simulink model "UAV_Hover_Sim"  (R2025a)
settings: Solver=VariableStepAuto  StartTime=0.0  StopTime=inf  RelTol=1e-3
undefined symbols (not defined in the file): quad_m, W
libraries: aerolibanimutils x1, uavutilslib x1
settings Model: Creator=Aorus PC  LastModifiedBy=esmithzb
settings OptimizationCC: ReuseModelBlockBuffer=off
settings DebuggingCC: UnderspecifiedInitializationDetection=Classic  MergeDetectMultiDrivingBlocksExec=none
settings ModelReferenceCC: PropagateSignalLabelsOutOfModel=off
settings RTWCC: GPUComputeCapability=3.5

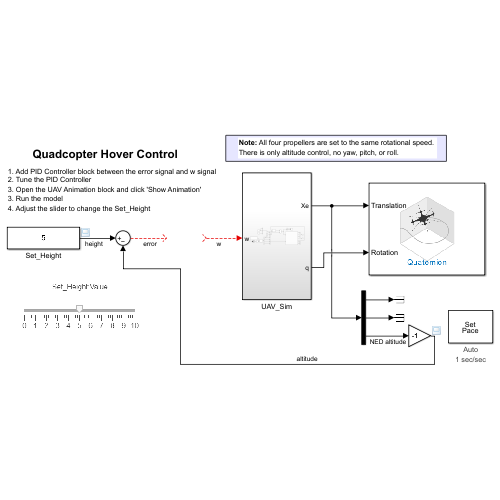
[thumbnail: Simulink's stored preview of the top-level diagram]
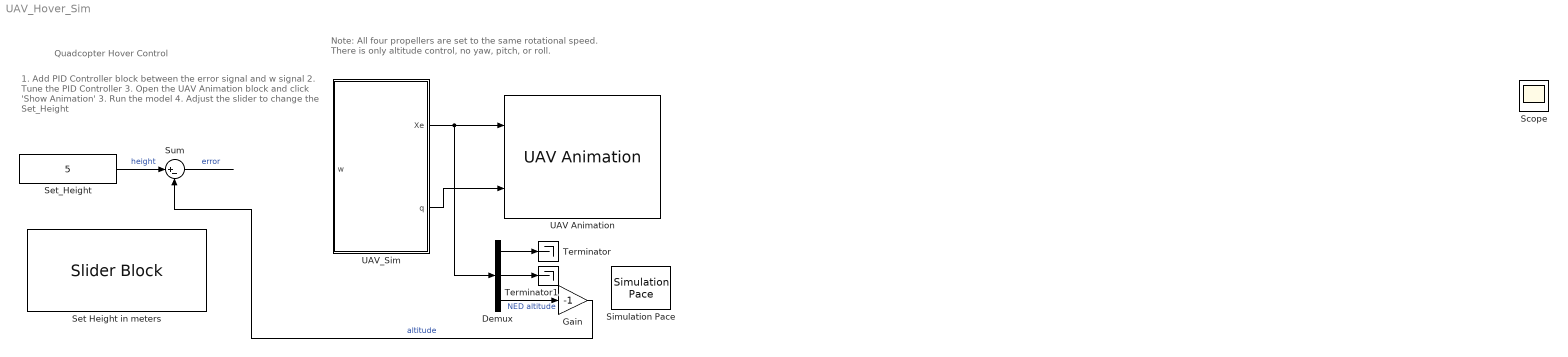
== system UAV_Hover_Sim ==
  note: Note: All four propellers are set to the same rotational speed.
      | There is only altitude control, no yaw, pitch, or roll.
  note: 1. Add PID Controller block between the error signal and w signal 2. Tune the PID Controller
      | 3. Open the UAV Animation block and click 'Show Animation'
      | 3. Run the model
      | 4. Adjust the slider to change the Set_Height
  note: Quadcopter Hover Control
  Demux : Demux  Outputs=3
  Gain : Gain  Gain=-1
  Set Height in meters : SliderBlock  ScaleMax=10  TickInterval=1
  Set_Height : Constant  Value=5
  Simulation Pace : aerolibanimutils/Simulation Pace  SimulationPace=1  SleepMode=Auto  OutputPaceError=off  SampleTime=1/30
  Sum : Sum  Inputs=|+-
  Terminator : Terminator
  Terminator1 : Terminator
  UAV Animation : uavutilslib/UAV Animation  NumUAV=1  DynamicUAVConfig=off  UAVType=Multirotor  UAVSize=4  UAVColor=[1 0 0]  UAVTrajectoryAlpha=1  InertialZDirection=Down  RotationFormat=Quaternion  DrawMarkers=off  SampleTime=-1
  UAV_Sim : Subsystem
  Scope : Scope
      settings: TimeSpan=20  ActiveDisplayYMinimum=0  ActiveDisplayYMaximum=12  YLabel=Altitude (m)
  wires:
  UAV_Sim/1(Xe) -> Demux/1, UAV Animation/1
  UAV_Sim/2(q) -> UAV Animation/2
  Demux/1 -> Terminator/1
  Demux/2 -> Terminator1/1
  Gain/1 -> Sum/2  "altitude"
  Set_Height/1 -> Sum/1  "height"
  Demux/3 -> Gain/1  "NED altitude"
  ? -> UAV_Sim/1(w)  "w"
  Sum/1 -> ?  "error"

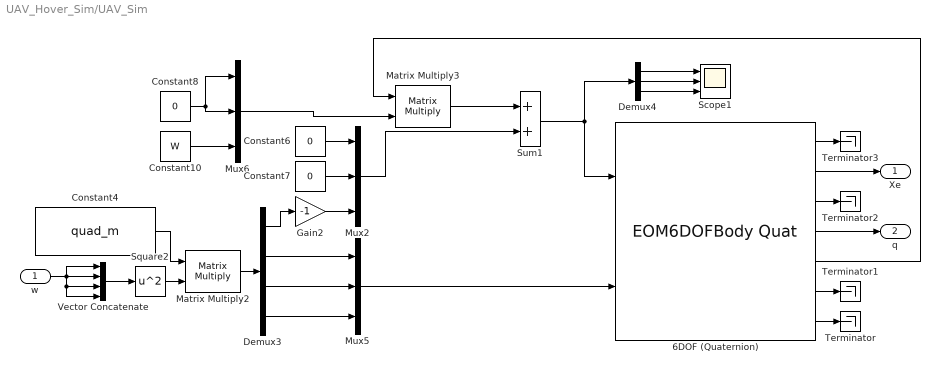
== system UAV_Hover_Sim/UAV_Sim ==
  w : Inport
  6DOF (Quaternion) : EOM6DOFBodyQuat
  Constant10 : Constant  Value=W
  Constant4 : Constant  Value=quad_m
  Constant6 : Constant  Value=0
  Constant7 : Constant  Value=0
  Constant8 : Constant  Value=0
  Demux3 : Demux
  Demux4 : Demux  Outputs=3
  Gain2 : Gain  Gain=-1
  Matrix Multiply2 : Product  Multiplication=Matrix(*)
  Matrix Multiply3 : Product  Multiplication=Matrix(*)
  Mux2 : Mux  Inputs=3
  Mux5 : Mux  Inputs=3
  Mux6 : Mux  Inputs=3
  Scope1 : Scope  NumInputPorts=3
      settings: ActiveDisplayYMinimum=-7E-15  ActiveDisplayYMaximum=8E-16  DataLoggingVariableName=ScopeData2
  Square2 : Math  Operator=square
  Sum1 : Sum
  Terminator{,1..3} (4 alike) : Terminator
  Vector Concatenate : Concatenate  NumInputs=4
  Xe : Outport
  q : Outport  Port=2
  wires:
  Mux2/1 -> Sum1/2
  Matrix Multiply3/1 -> Sum1/1
  Demux4/1 -> Scope1/1
  Mux6/1 -> Matrix Multiply3/2
  Constant10/1 -> Mux6/3
  Sum1/1 -> 6DOF (Quaternion)/1, Demux4/1
  Demux4/2 -> Scope1/2
  Constant4/1 -> Matrix Multiply2/1
  Demux3/1 -> Gain2/1
  Square2/1 -> Matrix Multiply2/2
  Matrix Multiply2/1 -> Demux3/1
  Demux3/2 -> Mux5/1
  Demux3/3 -> Mux5/2
  Demux3/4 -> Mux5/3
  Constant8/1 -> Mux6/2, Mux6/1
  Constant6/1 -> Mux2/1
  Constant7/1 -> Mux2/2
  Gain2/1 -> Mux2/3
  Demux4/3 -> Scope1/3
  w/1 -> Vector Concatenate/4, Vector Concatenate/3, Vector Concatenate/1, Vector Concatenate/2
  6DOF (Quaternion)/4 -> q/1
  6DOF (Quaternion)/5 -> Matrix Multiply3/1
  6DOF (Quaternion)/2 -> Xe/1
  Vector Concatenate/1 -> Square2/1
  Mux5/1 -> 6DOF (Quaternion)/2
  6DOF (Quaternion)/7 -> Terminator/1
  6DOF (Quaternion)/6 -> Terminator1/1
  6DOF (Quaternion)/3 -> Terminator2/1
  6DOF (Quaternion)/1 -> Terminator3/1
